simulink model "zcu216_tut_rfdc"  (R2019a)
settings: Solver=VariableStepDiscrete  StartTime=0.0  StopTime=10.0  RelTol=1e-3
undefined symbols (not defined in the file): es1, I, Q
libraries: xbsIndex_r4 x206, xps_library x3, casper_library_misc x1
(part 1 of 4)
settings Model: Creator=mcb  LastModifiedBy=mcb
settings OptimizationCC: DefaultParameterBehavior=Inlined

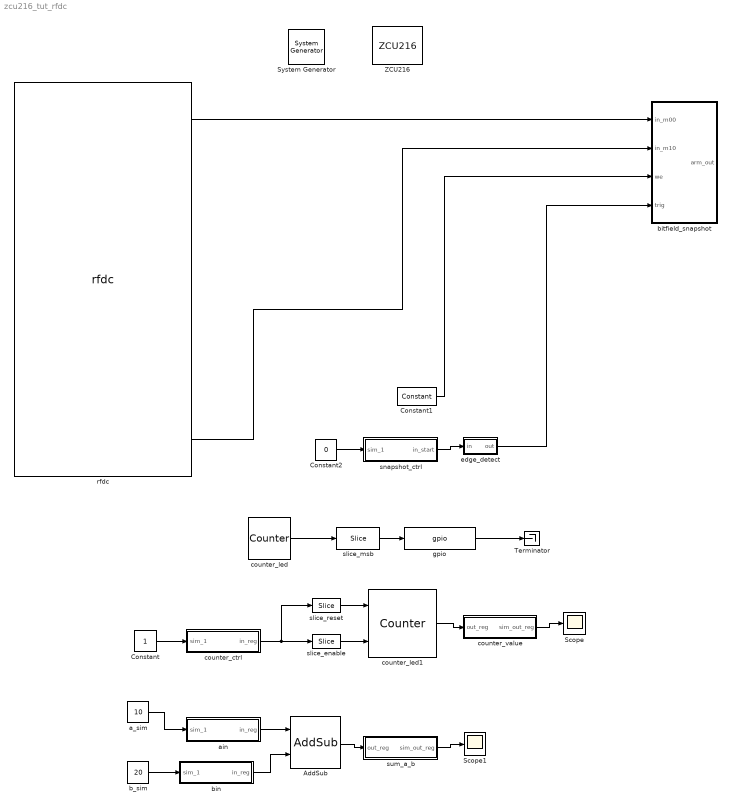
== system zcu216_tut_rfdc ==
  " System Generator" : xbsIndex_r4/ System Generator  Tag=genX  xilinxfamily=zynquplusRFSOCes1  part=xczu49dr  speed=-2-e-es1  package=ffvf1760  synthesis_tool=XST  clock_wrapper=Clock Enables  directory=/home/mcb/git/casper/tutorials_devel/rfsoc/tut_rfdc/zcu216_tut_rfdc/sysgen  proj_type=Vivado  Synth_file=Vivado Synthesis Defaults  Impl_file=Vivado Implementation Defaults  testbench=off  simulink_period=1  sysclk_period=4  dcm_input_clock_period=10  incr_netlist=off  trim_vbits=Everywhere in SubSystem  dbl_ovrd=According to Block Masks  core_generation=According to Block Masks  run_coregen=off  deprecated_control=off  eval_field=0  block_type=sysgen
  AddSub : xbsIndex_r4/AddSub  mode=Addition  use_carryin=off  use_carryout=off  en=off  latency=0  precision=User Defined  arith_type=Unsigned  n_bits=32  bin_pt=0  quantization=Truncate  overflow=Saturate  use_behavioral_HDL=off  hw_selection=Fabric  pipelined=off  dbl_ovrd=off  block_type=addsub
  Constant : Constant
  Constant1 : xbsIndex_r4/Constant  const=1.0  gui_display_data_type=Boolean  arith_type=Boolean  n_bits=16  bin_pt=14  preci_type=Single  exp_width=8  frac_width=24  explicit_period=on  period=1  equ=P=C  opselect=C  inp2=PCIN>>17  opr=+  inp1=P  carry=CIN  dbl_ovrd=off  block_type=constant
  Constant2 : Constant  Value=0
  Scope : Scope
  Scope1 : Scope
  Terminator : Terminator
  ZCU216 : xps_library/Platforms/ZCU216  Tag=xps:xsg  hw_sys=ZCU216:xczu49dr  clk_src=adc_clk  clk_rate=250  pl_clk_rate=125  sample_period=1  synthesis_tool=XST
      settings: SourceProductName=CASPER XPS Blockset
  a_sim : Constant  Value=10
  ain : Subsystem  Tag=xps:sw_reg  AncestorBlock=xps_library/Memory/software_register  mask(swreg){io_dir=From Processor, io_delay=0, init_val=0, sample_period=1, names=reg, bitwidths=32, bin_pts=0, arith_types=0, sim_port=on, show_format=off}
      mask prompts: io_dir "I/O direction"; io_delay "I/O delay"; init_val "Initial Value"; sample_period "Sample period"; names "Bitfield names [msb...lsb]"; bitwidths "Bitfield widths"; bin_pts "Bitfield binary pts"; arith_types "Bitfield types, ufix=0, fix=1, bool=2"; sim_port "Provide sim input/output?"; show_format "Print format string?"
      mask help: A 32-bit software-accessible register. Can be divided into bitfields of varying widths and types using the fields in the block mask.
      mask init:
      | swreg_init(gcb)
      settings: AttributesFormatString=1input
      mask TypeOptions io_dir: To Processor | From Processor
      mask Callback io_dir:
      | mask_enables = get_param(gcb, 'MaskEnables');
      | mask_names = get_param(gcb, 'MaskNames');
      | if strcmp(get_param(gcb, 'io_dir'), 'To Processor'),
      |     mask_enables{ismember(mask_names, 'sample_period')} = 'off';
      | else
      |     mask_enables{ismember(mask_names, 'sample_period')} = 'on';
      | end
      | set_param(gcb, 'MaskEnables', mask_enables);
      mask DialogControl ParameterTabVar0 Prompt: Setup
  b_sim : Constant  Value=20
  bin : Subsystem  Tag=xps:sw_reg  AncestorBlock=xps_library/Memory/software_register  mask(swreg){io_dir=From Processor, io_delay=0, init_val=0, sample_period=1, names=reg, bitwidths=32, bin_pts=0, arith_types=0, sim_port=on, show_format=off}
      mask prompts: io_dir "I/O direction"; io_delay "I/O delay"; init_val "Initial Value"; sample_period "Sample period"; names "Bitfield names [msb...lsb]"; bitwidths "Bitfield widths"; bin_pts "Bitfield binary pts"; arith_types "Bitfield types, ufix=0, fix=1, bool=2"; sim_port "Provide sim input/output?"; show_format "Print format string?"
      mask help: A 32-bit software-accessible register. Can be divided into bitfields of varying widths and types using the fields in the block mask.
      mask init:
      | swreg_init(gcb)
      settings: AttributesFormatString=1input
      mask TypeOptions io_dir: To Processor | From Processor
      mask Callback io_dir:
      | mask_enables = get_param(gcb, 'MaskEnables');
      | mask_names = get_param(gcb, 'MaskNames');
      | if strcmp(get_param(gcb, 'io_dir'), 'To Processor'),
      |     mask_enables{ismember(mask_names, 'sample_period')} = 'off';
      | else
      |     mask_enables{ismember(mask_names, 'sample_period')} = 'on';
      | end
      | set_param(gcb, 'MaskEnables', mask_enables);
      mask DialogControl ParameterTabVar0 Prompt: Setup
  bitfield_snapshot : Subsystem  Tag=casper:bitsnap  AncestorBlock=casper_library_scopes/bitfield_snapshot  mask(bitsnap){io_names=[m00 m10], io_widths=[64 64], io_bps=[0 0], io_types=[1 1], show_format=on, snap_storage=bram, snap_dram_dimm=2, snap_dram_clock=250, snap_nsamples=14, snap_data_width=128, snap_offset=off, snap_circap=off, snap_value=off, snap_ext_arm=off, snap_ext_circ=off, snap_provide_outputs=on, snap_use_dsp48=on, snap_delay=2, extra_names=[c d], extra_widths=[30 2], extra_bps=[0 0], extra_types=[0 0]}
      mask prompts: io_names "Names [msb...lsb]"; io_widths "Bitwidths [msb...lsb]"; io_bps "Binary pts [msb...lsb]"; io_types "Data types [msb...lsb], ufix=0, fix=1, bool=2"; show_format "Print format string?"; snap_storage "Storage medium"; snap_dram_dimm "DRAM dimm"; snap_dram_clock "DRAM clock rate"; snap_nsamples "Number of Samples (2^?)"; snap_data_width "Data width"; snap_offset "Start delay support"; snap_circap "Circular capture support"; snap_value "Extra value capture support"; snap_ext_arm "External arm support"; snap_ext_circ "External circular capture support"; snap_provide_outputs "Provide outputs"; snap_use_dsp48 "Use DSP48s to implement counters"; snap_delay "Pre-snapshot delay"; extra_names "Names [msb...lsb]"; extra_widths "Widths [msb...lsb]"; extra_bps "Binary pts [msb...lsb]"; extra_types "Data types [msb...lsb], ufix=0, fix=1, bool=2"
      mask help:
      | A wrapped snapshot block. Allows specification of inputs to a snapblock word so the toolflow can automatically set up the scope.
      | See documentation for snapshot for explanation of parameters.
      mask init:
      | bitsnap_init(gcb);
      settings: AttributesFormatString=|
      | snap(2):f64.0,f64.0 = 128 bits\n128 wide, 16384 deep
      | debugID: 51089287
      mask TypeOptions snap_storage: bram | dram
      mask Callback snap_storage: bitsnap_callback();
      mask TypeOptions snap_dram_dimm: 1 | 2 | 3 | 4
      mask TypeOptions snap_dram_clock: 200 | 250 | 266 | 300 | 333
      mask TypeOptions snap_data_width: 8 | 16 | 32 | 64 | 128
      mask Callback snap_value: bitsnap_callback();
      mask Callback snap_ext_arm: bitsnap_callback();
      mask Callback snap_ext_circ: bitsnap_callback();
      mask Callback snap_provide_outputs: bitsnap_callback();
      mask DialogControl ParameterTabVar0 Prompt: Inputs
      mask DialogControl ParameterTabVar01 Prompt: Snapshot
      mask DialogControl ParameterTabVar012 Prompt: Extra Value
  counter_ctrl : Subsystem  Tag=xps:sw_reg  AncestorBlock=xps_library/Memory/software_register  mask(swreg){io_dir=From Processor, io_delay=0, init_val=0, sample_period=1, names=reg, bitwidths=32, bin_pts=0, arith_types=0, sim_port=on, show_format=off}
      mask prompts: io_dir "I/O direction"; io_delay "I/O delay"; init_val "Initial Value"; sample_period "Sample period"; names "Bitfield names [msb...lsb]"; bitwidths "Bitfield widths"; bin_pts "Bitfield binary pts"; arith_types "Bitfield types, ufix=0, fix=1, bool=2"; sim_port "Provide sim input/output?"; show_format "Print format string?"
      mask help: A 32-bit software-accessible register. Can be divided into bitfields of varying widths and types using the fields in the block mask.
      mask init:
      | swreg_init(gcb)
      settings: AttributesFormatString=1input
      mask TypeOptions io_dir: To Processor | From Processor
      mask Callback io_dir:
      | mask_enables = get_param(gcb, 'MaskEnables');
      | mask_names = get_param(gcb, 'MaskNames');
      | if strcmp(get_param(gcb, 'io_dir'), 'To Processor'),
      |     mask_enables{ismember(mask_names, 'sample_period')} = 'off';
      | else
      |     mask_enables{ismember(mask_names, 'sample_period')} = 'on';
      | end
      | set_param(gcb, 'MaskEnables', mask_enables);
      mask DialogControl ParameterTabVar0 Prompt: Setup
  counter_led : xbsIndex_r4/Counter  cnt_type=Free Running  cnt_to=Inf  operation=Up  start_count=0  cnt_by_val=1  arith_type=Unsigned  n_bits=28  bin_pt=0  load_pin=off  rst=off  en=off  explicit_period=on  period=1  use_behavioral_HDL=off  implementation=Fabric  dbl_ovrd=off  block_type=counter
  counter_led1 : xbsIndex_r4/Counter  cnt_type=Free Running  cnt_to=Inf  operation=Up  start_count=0  cnt_by_val=1  arith_type=Unsigned  n_bits=32  bin_pt=0  load_pin=off  rst=on  en=on  explicit_period=on  period=1  use_behavioral_HDL=off  implementation=Fabric  dbl_ovrd=off  block_type=counter
  counter_value : Subsystem  Tag=xps:sw_reg  AncestorBlock=xps_library/Memory/software_register  mask(swreg){io_dir=To Processor, io_delay=0, init_val=0, sample_period=1, names=reg, bitwidths=32, bin_pts=0, arith_types=0, sim_port=on, show_format=off}
      mask prompts: io_dir "I/O direction"; io_delay "I/O delay"; init_val "Initial Value"; sample_period "Sample period"; names "Bitfield names [msb...lsb]"; bitwidths "Bitfield widths"; bin_pts "Bitfield binary pts"; arith_types "Bitfield types, ufix=0, fix=1, bool=2"; sim_port "Provide sim input/output?"; show_format "Print format string?"
      mask help: A 32-bit software-accessible register. Can be divided into bitfields of varying widths and types using the fields in the block mask.
      mask init:
      | swreg_init(gcb)
      settings: AttributesFormatString=1output
      mask TypeOptions io_dir: To Processor | From Processor
      mask Callback io_dir:
      | mask_enables = get_param(gcb, 'MaskEnables');
      | mask_names = get_param(gcb, 'MaskNames');
      | if strcmp(get_param(gcb, 'io_dir'), 'To Processor'),
      |     mask_enables{ismember(mask_names, 'sample_period')} = 'off';
      | else
      |     mask_enables{ismember(mask_names, 'sample_period')} = 'on';
      | end
      | set_param(gcb, 'MaskEnables', mask_enables);
      mask DialogControl ParameterTabVar0 Prompt: Setup
  edge_detect : Subsystem  AncestorBlock=casper_library_misc/edge_detect  mask(edge_detect){edge=Rising, polarity=Active High, x_in=[0 0.08 0.08 0.16 0.16 0.24 0.24 0.32 0.32 0.4], y_in=[-1 -1  1  1  1  1  1  1  1  1], x_out=[0.6 0.68 0.68 0.76 0.76 0.84 0.84 0.92 0.92 1], y_out=[-1 -1  1  1 -1 -1 -1 -1 -1 -1]}
      mask prompts: edge "Edge Type"; polarity "Output Polarity"; x_in "Input X Positions"; y_in "Input Y Positions"; x_out "Output X Positions"; y_out "Output Y Positions"
      mask help: Output is active for one-cycle after each edge of the specified type (i.e. rising, falling or both).
      mask init:
      | edge_detect_init(gcb,...
      |     'edge',edge,...
      |     'polarity',polarity,...
      |     'x_in',x_in,...
      |     'x_out',x_out,...
      |     'y_in',y_in,...
      |     'y_out',y_out);
      | 
      | x_in_num=str2num(getfield(getfield(get_param(gcb,'UserData'),'parameters'),'x_in'));
      | x_out_num=str2num(getfield(getfield(get_param(gcb,'UserData'),'parameters'),'x_out'));
      | y_in_num=str2num(getfield(getfield(get_param(gcb,'UserData'),'parameters'),'y_in'));
      | y_out_num=str2num(getfield(getfield(get_param(gcb,'UserData'),'parameters'),'y_out'));
      settings: AttributesFormatString=|
      | rising edges
      | active high
      mask Help: Output is active for one-cycle after each edge of the specified type (i.e. rising, falling, or both).  Latency is zero.
      mask TypeOptions edge: Rising | Falling | Both
      mask TypeOptions polarity: Active High | Active Low
      mask Display:
      | plot(x_in_num,0.5+y_in_num*0.2);
      | plot(x_out_num,0.5+y_out_num*0.2);
  gpio : xps_library/IO/gpio  Tag=xps:gpio  io_group_params_forwarded=on  io_group=ROACH2:led  io_group_real=led  io_group_custom=0  io_dir=out  arith_type=Boolean  bitwidth=1  bin_pt=0  bit_index=0  sample_period=1  use_single_ended=off  use_ddr=off  reg_iob=on  reg_clk_phase=0  termination=None
      settings: SourceProductName=CASPER XPS Blockset
  rfdc : xps_library/ADCs/rfdc  Tag=xps:rfdc  forceredraw=0  maskopening=1  runinit=1  Tile224_enable=on  t224_enable_mts=off  t224_sample_rate=2000  t224_clk_out=125  t224_enable_pll=on  t224_ref_clk=250  t224_QT_adc0_enable=on  t224_QT_adc0_digital_output=I/Q  t224_QT_adc0_dec_mode=4x  t224_QT_adc0_sample_per_cycle=4  t224_QT_adc0_req_axis_clk=250  t224_QT_adc0_mixer_type=Fine  t224_QT_adc0_mixer_mode=Real -> I/Q  t224_QT_adc0_nco_freq=0.5  t224_QT_adc0_nco_phase=0  t224_QT_adc0_coarse_freq=0  t224_QT_adc0_nyquist_zone=Zone 2  t224_QT_adc0_cal_mode=Mode 2  t224_QT_adc1_enable=off  t224_QT_adc1_digital_output=I/Q  t224_QT_adc1_dec_mode=4x  t224_QT_adc1_sample_per_cycle=4  t224_QT_adc1_req_axis_clk=250  t224_QT_adc1_mixer_type=Fine  t224_QT_adc1_mixer_mode=Real -> I/Q  t224_QT_adc1_nco_freq=0  t224_QT_adc1_nco_phase=0  t224_QT_adc1_coarse_freq=0  t224_QT_adc1_nyquist_zone=Zone 1  t224_QT_adc1_cal_mode=Mode 2  t224_QT_adc2_enable=on  t224_QT_adc2_digital_output=I/Q  t224_QT_adc2_dec_mode=4x  t224_QT_adc2_sample_per_cycle=4  t224_QT_adc2_req_axis_clk=250  t224_QT_adc2_mixer_type=Fine  t224_QT_adc2_mixer_mode=Real -> I/Q  t224_QT_adc2_nco_freq=0.5  t224_QT_adc2_nco_phase=0  t224_QT_adc2_coarse_freq=0  t224_QT_adc2_nyquist_zone=Zone 2  t224_QT_adc2_cal_mode=Mode 2  t224_QT_adc3_enable=off  t224_QT_adc3_digital_output=I/Q  t224_QT_adc3_dec_mode=4x  t224_QT_adc3_sample_per_cycle=4  t224_QT_adc3_req_axis_clk=250  t224_QT_adc3_mixer_type=Fine  t224_QT_adc3_mixer_mode=Real -> I/Q  t224_QT_adc3_nco_freq=0  t224_QT_adc3_nco_phase=0  t224_QT_adc3_coarse_freq=0  t224_QT_adc3_nyquist_zone=Zone 1  t224_QT_adc3_cal_mode=Mode 2  t224_DT_adc0_enable=on  t224_DT_adc0_digital_output=Real  t224_DT_adc0_dec_mode=2x  t224_DT_adc0_sample_per_cycle=8  t224_DT_adc0_req_axis_clk=125  t224_DT_adc0_mixer_type=Bypassed  t224_DT_adc0_mixer_mode=Real -> Real  t224_DT_adc0_nco_freq=0  t224_DT_adc0_nco_phase=0  t224_DT_adc0_coarse_freq=0  t224_DT_adc0_nyquist_zone=Zone 1  t224_DT_adc0_cal_mode=Mode 2  t224_DT_adc1_enable=on  t224_DT_adc1_digital_output=Real  t224_DT_adc1_dec_mode=2x  t224_DT_adc1_sample_per_cycle=8  t224_DT_adc1_req_axis_clk=125  t224_DT_adc1_mixer_type=Bypassed  t224_DT_adc1_mixer_mode=Real -> Real  t224_DT_adc1_nco_freq=0  t224_DT_adc1_nco_phase=0  t224_DT_adc1_coarse_freq=0  t224_DT_adc1_nyquist_zone=Zone 1  t224_DT_adc1_cal_mode=Mode 2  Tile225_enable=on  t225_enable_mts=off  t225_sample_rate=2000  t225_clk_out=125  t225_enable_pll=on  t225_ref_clk=250  t225_QT_adc0_enable=on  t225_QT_adc0_digital_output=I/Q  t225_QT_adc0_dec_mode=4x  t225_QT_adc0_sample_per_cycle=4  t225_QT_adc0_req_axis_clk=250  t225_QT_adc0_mixer_type=Bypassed  t225_QT_adc0_mixer_mode=Real -> Real  t225_QT_adc0_nco_freq=0.5  t225_QT_adc0_nco_phase=0  t225_QT_adc0_coarse_freq=0  t225_QT_adc0_nyquist_zone=Zone 2  t225_QT_adc0_cal_mode=Mode 2  t225_QT_adc1_enable=off  t225_QT_adc1_digital_output=Real  t225_QT_adc1_dec_mode=4x  t225_QT_adc1_sample_per_cycle=2  t225_QT_adc1_req_axis_clk=250  t225_QT_adc1_mixer_type=Bypassed  t225_QT_adc1_mixer_mode=Real -> Real  t225_QT_adc1_nco_freq=0  t225_QT_adc1_nco_phase=0  t225_QT_adc1_coarse_freq=0  t225_QT_adc1_nyquist_zone=Zone 1  t225_QT_adc1_cal_mode=Mode 2  t225_QT_adc2_enable=on  t225_QT_adc2_digital_output=I/Q  t225_QT_adc2_dec_mode=4x  t225_QT_adc2_sample_per_cycle=4  t225_QT_adc2_req_axis_clk=250  t225_QT_adc2_mixer_type=Bypassed  t225_QT_adc2_mixer_mode=Real -> Real  t225_QT_adc2_nco_freq=0.5  t225_QT_adc2_nco_phase=0  t225_QT_adc2_coarse_freq=0  t225_QT_adc2_nyquist_zone=Zone 2  t225_QT_adc2_cal_mode=Mode 2  t225_QT_adc3_enable=off  t225_QT_adc3_digital_output=Real  t225_QT_adc3_dec_mode=4x  t225_QT_adc3_sample_per_cycle=2  t225_QT_adc3_req_axis_clk=250  t225_QT_adc3_mixer_type=Bypassed  t225_QT_adc3_mixer_mode=Real -> Real  t225_QT_adc3_nco_freq=0  t225_QT_adc3_nco_phase=0  t225_QT_adc3_coarse_freq=0  t225_QT_adc3_nyquist_zone=Zone 1  t225_QT_adc3_cal_mode=Mode 2  t225_DT_adc0_enable=on  t225_DT_adc0_digital_output=Real  t225_DT_adc0_dec_mode=2x  t225_DT_adc0_sample_per_cycle=8  t225_DT_adc0_req_axis_clk=125  t225_DT_adc0_mixer_type=Bypassed  t225_DT_adc0_mixer_mode=Real -> Real  t225_DT_adc0_nco_freq=0  t225_DT_adc0_nco_phase=0  t225_DT_adc0_coarse_freq=0  t225_DT_adc0_nyquist_zone=Zone 1  t225_DT_adc0_cal_mode=Mode 2  t225_DT_adc1_enable=on  t225_DT_adc1_digital_output=Real  t225_DT_adc1_dec_mode=2x  t225_DT_adc1_sample_per_cycle=8  t225_DT_adc1_req_axis_clk=125  t225_DT_adc1_mixer_type=Bypassed  t225_DT_adc1_mixer_mode=Real -> Real  t225_DT_adc1_nco_freq=0  t225_DT_adc1_nco_phase=0  t225_DT_adc1_coarse_freq=0  t225_DT_adc1_nyquist_zone=Zone 1  t225_DT_adc1_cal_mode=Mode 2  Tile226_enable=on  t226_enable_mts=off  t226_sample_rate=2000  t226_clk_out=125  t226_enable_pll=on  t226_ref_clk=250  t226_QT_adc0_enable=on  t226_QT_adc0_digital_output=I/Q  t226_QT_adc0_dec_mode=4x  t226_QT_adc0_sample_per_cycle=4  t226_QT_adc0_req_axis_clk=250  t226_QT_adc0_mixer_type=Bypassed  t226_QT_adc0_mixer_mode=Real -> Real  t226_QT_adc0_nco_freq=0.5  t226_QT_adc0_nco_phase=0  t226_QT_adc0_coarse_freq=0  t226_QT_adc0_nyquist_zone=Zone 2  t226_QT_adc0_cal_mode=Mode 2  t226_QT_adc1_enable=off  t226_QT_adc1_digital_output=Real  t226_QT_adc1_dec_mode=4x  t226_QT_adc1_sample_per_cycle=2  t226_QT_adc1_req_axis_clk=250  t226_QT_adc1_mixer_type=Bypassed  t226_QT_adc1_mixer_mode=Real -> Real  t226_QT_adc1_nco_freq=0  t226_QT_adc1_nco_phase=0  t226_QT_adc1_coarse_freq=0  t226_QT_adc1_nyquist_zone=Zone 1  t226_QT_adc1_cal_mode=Mode 2  t226_QT_adc2_enable=off  t226_QT_adc2_digital_output=Real  t226_QT_adc2_dec_mode=4x  t226_QT_adc2_sample_per_cycle=2  t226_QT_adc2_req_axis_clk=250  t226_QT_adc2_mixer_type=Bypassed  t226_QT_adc2_mixer_mode=Real -> Real  t226_QT_adc2_nco_freq=0  t226_QT_adc2_nco_phase=0  t226_QT_adc2_coarse_freq=0  t226_QT_adc2_nyquist_zone=Zone 1  t226_QT_adc2_cal_mode=Mode 2  t226_QT_adc3_enable=off  t226_QT_adc3_digital_output=Real  t226_QT_adc3_dec_mode=4x  t226_QT_adc3_sample_per_cycle=2  t226_QT_adc3_req_axis_clk=250  t226_QT_adc3_mixer_type=Bypassed  t226_QT_adc3_mixer_mode=Real -> Real  t226_QT_adc3_nco_freq=0  t226_QT_adc3_nco_phase=0  t226_QT_adc3_coarse_freq=0  t226_QT_adc3_nyquist_zone=Zone 1  t226_QT_adc3_cal_mode=Mode 2  t226_DT_adc0_enable=on  t226_DT_adc0_digital_output=Real  t226_DT_adc0_dec_mode=2x  t226_DT_adc0_sample_per_cycle=8  t226_DT_adc0_req_axis_clk=125  t226_DT_adc0_mixer_type=Bypassed  t226_DT_adc0_mixer_mode=Real -> Real  t226_DT_adc0_nco_freq=0  t226_DT_adc0_nco_phase=0  t226_DT_adc0_coarse_freq=0  t226_DT_adc0_nyquist_zone=Zone 1  t226_DT_adc0_cal_mode=Mode 2  t226_DT_adc1_enable=on  t226_DT_adc1_digital_output=Real  t226_DT_adc1_dec_mode=2x  t226_DT_adc1_sample_per_cycle=8  t226_DT_adc1_req_axis_clk=125  t226_DT_adc1_mixer_type=Bypassed  t226_DT_adc1_mixer_mode=Real -> Real  t226_DT_adc1_nco_freq=0  t226_DT_adc1_nco_phase=0  t226_DT_adc1_coarse_freq=0  t226_DT_adc1_nyquist_zone=Zone 1  t226_DT_adc1_cal_mode=Mode 2  Tile227_enable=on  t227_enable_mts=off  t227_sample_rate=2000  t227_clk_out=125  t227_enable_pll=on  t227_ref_clk=250  t227_QT_adc0_enable=on  t227_QT_adc0_digital_output=I/Q  t227_QT_adc0_dec_mode=4x  t227_QT_adc0_sample_per_cycle=4  t227_QT_adc0_req_axis_clk=250  t227_QT_adc0_mixer_type=Bypassed  t227_QT_adc0_mixer_mode=Real -> Real  t227_QT_adc0_nco_freq=0.5  t227_QT_adc0_nco_phase=0  t227_QT_adc0_coarse_freq=0  t227_QT_adc0_nyquist_zone=Zone 2  t227_QT_adc0_cal_mode=Mode 2  t227_QT_adc1_enable=off  t227_QT_adc1_digital_output=Real  t227_QT_adc1_dec_mode=4x  t227_QT_adc1_sample_per_cycle=2  t227_QT_adc1_req_axis_clk=250  t227_QT_adc1_mixer_type=Bypassed  t227_QT_adc1_mixer_mode=Real -> Real  t227_QT_adc1_nco_freq=0  t227_QT_adc1_nco_phase=0  t227_QT_adc1_coarse_freq=0  t227_QT_adc1_nyquist_zone=Zone 1  t227_QT_adc1_cal_mode=Mode 2  t227_QT_adc2_enable=off  t227_QT_adc2_digital_output=Real  t227_QT_adc2_dec_mode=4x  t227_QT_adc2_sample_per_cycle=2  t227_QT_adc2_req_axis_clk=250  t227_QT_adc2_mixer_type=Bypassed  t227_QT_adc2_mixer_mode=Real -> Real  t227_QT_adc2_nco_freq=0  t227_QT_adc2_nco_phase=0  t227_QT_adc2_coarse_freq=0  t227_QT_adc2_nyquist_zone=Zone 1  t227_QT_adc2_cal_mode=Mode 2  t227_QT_adc3_enable=off  t227_QT_adc3_digital_output=Real  t227_QT_adc3_dec_mode=4x  t227_QT_adc3_sample_per_cycle=2  t227_QT_adc3_req_axis_clk=250  t227_QT_adc3_mixer_type=Bypassed  t227_QT_adc3_mixer_mode=Real -> Real  t227_QT_adc3_nco_freq=0  t227_QT_adc3_nco_phase=0  t227_QT_adc3_coarse_freq=0  t227_QT_adc3_nyquist_zone=Zone 1  t227_QT_adc3_cal_mode=Mode 2  t227_DT_adc0_enable=on  t227_DT_adc0_digital_output=Real  t227_DT_adc0_dec_mode=2x  t227_DT_adc0_sample_per_cycle=8  t227_DT_adc0_req_axis_clk=125  t227_DT_adc0_mixer_type=Bypassed  t227_DT_adc0_mixer_mode=Real -> Real  t227_DT_adc0_nco_freq=0  t227_DT_adc0_nco_phase=0  t227_DT_adc0_coarse_freq=0  t227_DT_adc0_nyquist_zone=Zone 1  t227_DT_adc0_cal_mode=Mode 2  t227_DT_adc1_enable=on  t227_DT_adc1_digital_output=Real  t227_DT_adc1_dec_mode=2x  t227_DT_adc1_sample_per_cycle=8  t227_DT_adc1_req_axis_clk=125  t227_DT_adc1_mixer_type=Bypassed  t227_DT_adc1_mixer_mode=Real -> Real  t227_DT_adc1_nco_freq=0  t227_DT_adc1_nco_phase=0  t227_DT_adc1_coarse_freq=0  t227_DT_adc1_nyquist_zone=Zone 1  t227_DT_adc1_cal_mode=Mode 2  Tile228_enable=off  t228_enable_mts=off  t228_sample_rate=2000  t228_clk_out=125  t228_enable_pll=on  t228_ref_clk=250  t228_output_power=20  t228_QT_dac0_enable=off  t228_QT_dac0_analog_output=Real  t228_QT_dac0_inter_mode=4x  t228_QT_dac0_sample_per_cycle=2  t228_QT_dac0_req_axis_clk=250  t228_QT_dac0_datapath_mode=DUC 0 to Fs/2  t228_QT_dac0_mixer_type=Bypassed  t228_QT_dac0_mixer_mode=Real -> Real  t228_QT_dac0_nco_freq=0  t228_QT_dac0_nco_phase=0  t228_QT_dac0_coarse_freq=0  t228_QT_dac0_nyquist_zone=Zone 1  t228_QT_dac0_decode_mode=SNR Optimized  t228_QT_dac1_enable=off  t228_QT_dac1_analog_output=Real  t228_QT_dac1_inter_mode=4x  t228_QT_dac1_sample_per_cycle=2  t228_QT_dac1_req_axis_clk=250  t228_QT_dac1_datapath_mode=DUC 0 to Fs/2  t228_QT_dac1_mixer_type=Bypassed  t228_QT_dac1_mixer_mode=Real -> Real  t228_QT_dac1_nco_freq=0  t228_QT_dac1_nco_phase=0  t228_QT_dac1_coarse_freq=0  t228_QT_dac1_nyquist_zone=Zone 1  t228_QT_dac1_decode_mode=SNR Optimized  t228_QT_dac2_enable=off  t228_QT_dac2_analog_output=Real  t228_QT_dac2_inter_mode=4x  t228_QT_dac2_sample_per_cycle=2  t228_QT_dac2_req_axis_clk=250  t228_QT_dac2_datapath_mode=DUC 0 to Fs/2  t228_QT_dac2_mixer_type=Bypassed  t228_QT_dac2_mixer_mode=Real -> Real  t228_QT_dac2_nco_freq=0  t228_QT_dac2_nco_phase=0  t228_QT_dac2_coarse_freq=0  t228_QT_dac2_nyquist_zone=Zone 1  t228_QT_dac2_decode_mode=SNR Optimized  t228_QT_dac3_enable=off  t228_QT_dac3_analog_output=Real  t228_QT_dac3_inter_mode=4x  t228_QT_dac3_sample_per_cycle=2  t228_QT_dac3_req_axis_clk=250  t228_QT_dac3_datapath_mode=DUC 0 to Fs/2  t228_QT_dac3_mixer_type=Bypassed  t228_QT_dac3_mixer_mode=Real -> Real  t228_QT_dac3_nco_freq=0  t228_QT_dac3_nco_phase=0  t228_QT_dac3_coarse_freq=0  t228_QT_dac3_nyquist_zone=Zone 1  t228_QT_dac3_decode_mode=SNR Optimized  t228_DT_dac0_enable=on  t228_DT_dac0_analog_output=I/Q  t228_DT_dac0_inter_mode=2x  t228_DT_dac0_sample_per_cycle=8  t228_DT_dac0_req_axis_clk=125  t228_DT_dac0_mixer_type=Fine  t228_DT_dac0_mixer_mode=I/Q -> I/Q  t228_DT_dac0_nco_freq=0  t228_DT_dac0_nco_phase=0  t228_DT_dac0_coarse_freq=0  t228_DT_dac0_nyquist_zone=Zone 1  t228_DT_dac0_decode_mode=SNR Optimized  t228_DT_dac1_enable=on  t228_DT_dac1_analog_output=I/Q  t228_DT_dac1_inter_mode=2x  t228_DT_dac1_sample_per_cycle=8  t228_DT_dac1_req_axis_clk=125  t228_DT_dac1_mixer_type=Off  t228_DT_dac1_mixer_mode=Off  t228_DT_dac1_nco_freq=0  t228_DT_dac1_nco_phase=0  t228_DT_dac1_coarse_freq=0  t228_DT_dac1_nyquist_zone=Zone 1  t228_DT_dac1_decode_mode=SNR Optimized  t228_DT_dac2_enable=on  t228_DT_dac2_analog_output=Real  t228_DT_dac2_inter_mode=2x  t228_DT_dac2_sample_per_cycle=8  t228_DT_dac2_req_axis_clk=125  t228_DT_dac2_mixer_type=Bypassed  t228_DT_dac2_mixer_mode=Real -> Real  t228_DT_dac2_nco_freq=0  t228_DT_dac2_nco_phase=0  t228_DT_dac2_coarse_freq=0  t228_DT_dac2_nyquist_zone=Zone 1  t228_DT_dac2_decode_mode=SNR Optimized  t228_DT_dac3_enable=off  t228_DT_dac3_analog_output=Real  t228_DT_dac3_inter_mode=2x  t228_DT_dac3_sample_per_cycle=8  t228_DT_dac3_req_axis_clk=125  t228_DT_dac3_mixer_type=Bypassed  t228_DT_dac3_mixer_mode=Real -> Real  t228_DT_dac3_nco_freq=0  t228_DT_dac3_nco_phase=0  t228_DT_dac3_coarse_freq=0  t228_DT_dac3_nyquist_zone=Zone 1  t228_DT_dac3_decode_mode=SNR Optimized  Tile229_enable=off  t229_enable_mts=off  t229_sample_rate=2000  t229_clk_out=125  t229_enable_pll=on  t229_ref_clk=250  t229_output_power=20  t229_QT_dac0_enable=off  t229_QT_dac0_analog_output=Real  t229_QT_dac0_inter_mode=4x  t229_QT_dac0_sample_per_cycle=2  t229_QT_dac0_req_axis_clk=250  t229_QT_dac0_datapath_mode=DUC 0 to Fs/2  t229_QT_dac0_mixer_type=Bypassed  t229_QT_dac0_mixer_mode=Real -> Real  t229_QT_dac0_nco_freq=0  t229_QT_dac0_nco_phase=0  t229_QT_dac0_coarse_freq=0  t229_QT_dac0_nyquist_zone=Zone 1  t229_QT_dac0_decode_mode=SNR Optimized  t229_QT_dac1_enable=off  t229_QT_dac1_analog_output=Real  t229_QT_dac1_inter_mode=4x  t229_QT_dac1_sample_per_cycle=2  t229_QT_dac1_req_axis_clk=250  t229_QT_dac1_datapath_mode=DUC 0 to Fs/2  t229_QT_dac1_mixer_type=Bypassed  t229_QT_dac1_mixer_mode=Real -> Real  t229_QT_dac1_nco_freq=0  t229_QT_dac1_nco_phase=0  t229_QT_dac1_coarse_freq=0  t229_QT_dac1_nyquist_zone=Zone 1  t229_QT_dac1_decode_mode=SNR Optimized  t229_QT_dac2_enable=off  t229_QT_dac2_analog_output=Real  t229_QT_dac2_inter_mode=4x  t229_QT_dac2_sample_per_cycle=2  t229_QT_dac2_req_axis_clk=250  t229_QT_dac2_datapath_mode=DUC 0 to Fs/2  t229_QT_dac2_mixer_type=Bypassed  t229_QT_dac2_mixer_mode=Real -> Real  t229_QT_dac2_nco_freq=0  t229_QT_dac2_nco_phase=0  t229_QT_dac2_coarse_freq=0  t229_QT_dac2_nyquist_zone=Zone 1  t229_QT_dac2_decode_mode=SNR Optimized  t229_QT_dac3_enable=off  t229_QT_dac3_analog_output=Real  t229_QT_dac3_inter_mode=4x  t229_QT_dac3_sample_per_cycle=2  t229_QT_dac3_req_axis_clk=250  t229_QT_dac3_datapath_mode=DUC 0 to Fs/2  t229_QT_dac3_mixer_type=Bypassed  t229_QT_dac3_mixer_mode=Real -> Real  t229_QT_dac3_nco_freq=0  t229_QT_dac3_nco_phase=0  t229_QT_dac3_coarse_freq=0  t229_QT_dac3_nyquist_zone=Zone 1  t229_QT_dac3_decode_mode=SNR Optimized  t229_DT_dac0_enable=off  t229_DT_dac0_analog_output=Real  t229_DT_dac0_inter_mode=2x  t229_DT_dac0_sample_per_cycle=8  t229_DT_dac0_req_axis_clk=125  t229_DT_dac0_mixer_type=Bypassed  t229_DT_dac0_mixer_mode=Real -> Real  t229_DT_dac0_nco_freq=0  t229_DT_dac0_nco_phase=0  t229_DT_dac0_coarse_freq=0  t229_DT_dac0_nyquist_zone=Zone 1  t229_DT_dac0_decode_mode=SNR Optimized  t229_DT_dac1_enable=off  t229_DT_dac1_analog_output=Real  t229_DT_dac1_inter_mode=2x  t229_DT_dac1_sample_per_cycle=8  t229_DT_dac1_req_axis_clk=125  t229_DT_dac1_mixer_type=Bypassed  t229_DT_dac1_mixer_mode=Real -> Real  t229_DT_dac1_nco_freq=0  t229_DT_dac1_nco_phase=0  t229_DT_dac1_coarse_freq=0  t229_DT_dac1_nyquist_zone=Zone 1  t229_DT_dac1_decode_mode=SNR Optimized  t229_DT_dac2_enable=off  t229_DT_dac2_analog_output=Real  t229_DT_dac2_inter_mode=2x  t229_DT_dac2_sample_per_cycle=8  t229_DT_dac2_req_axis_clk=125  t229_DT_dac2_mixer_type=Bypassed  t229_DT_dac2_mixer_mode=Real -> Real  t229_DT_dac2_nco_freq=0  t229_DT_dac2_nco_phase=0  t229_DT_dac2_coarse_freq=0  t229_DT_dac2_nyquist_zone=Zone 1  t229_DT_dac2_decode_mode=SNR Optimized  t229_DT_dac3_enable=off  t229_DT_dac3_analog_output=Real  t229_DT_dac3_inter_mode=2x  t229_DT_dac3_sample_per_cycle=8  t229_DT_dac3_req_axis_clk=125  t229_DT_dac3_mixer_type=Bypassed  t229_DT_dac3_mixer_mode=Real -> Real  t229_DT_dac3_nco_freq=0  t229_DT_dac3_nco_phase=0  t229_DT_dac3_coarse_freq=0  t229_DT_dac3_nyquist_zone=Zone 1  t229_DT_dac3_decode_mode=SNR Optimized  Tile230_enable=off  t230_enable_mts=off  t230_sample_rate=2000  t230_clk_out=125  t230_enable_pll=on  t230_ref_clk=250  t230_output_power=20  t230_QT_dac0_enable=off  t230_QT_dac0_analog_output=Real  t230_QT_dac0_inter_mode=4x  t230_QT_dac0_sample_per_cycle=2  t230_QT_dac0_req_axis_clk=250  t230_QT_dac0_datapath_mode=DUC 0 to Fs/2  t230_QT_dac0_mixer_type=Bypassed  t230_QT_dac0_mixer_mode=Real -> Real  t230_QT_dac0_nco_freq=0  t230_QT_dac0_nco_phase=0  t230_QT_dac0_coarse_freq=0  t230_QT_dac0_nyquist_zone=Zone 1  t230_QT_dac0_decode_mode=SNR Optimized  t230_QT_dac1_enable=off  t230_QT_dac1_analog_output=Real  t230_QT_dac1_inter_mode=4x  t230_QT_dac1_sample_per_cycle=2  t230_QT_dac1_req_axis_clk=250  t230_QT_dac1_datapath_mode=DUC 0 to Fs/2  t230_QT_dac1_mixer_type=Bypassed  t230_QT_dac1_mixer_mode=Real -> Real  t230_QT_dac1_nco_freq=0  t230_QT_dac1_nco_phase=0  t230_QT_dac1_coarse_freq=0  t230_QT_dac1_nyquist_zone=Zone 1  t230_QT_dac1_decode_mode=SNR Optimized  t230_QT_dac2_enable=off  t230_QT_dac2_analog_output=Real  t230_QT_dac2_inter_mode=4x  t230_QT_dac2_sample_per_cycle=2  t230_QT_dac2_req_axis_clk=250  t230_QT_dac2_datapath_mode=DUC 0 to Fs/2  t230_QT_dac2_mixer_type=Bypassed  t230_QT_dac2_mixer_mode=Real -> Real  t230_QT_dac2_nco_freq=0  t230_QT_dac2_nco_phase=0  t230_QT_dac2_coarse_freq=0  t230_QT_dac2_nyquist_zone=Zone 1  t230_QT_dac2_decode_mode=SNR Optimized  t230_QT_dac3_enable=off  t230_QT_dac3_analog_output=Real  t230_QT_dac3_inter_mode=4x  t230_QT_dac3_sample_per_cycle=2  t230_QT_dac3_req_axis_clk=250  t230_QT_dac3_datapath_mode=DUC 0 to Fs/2  t230_QT_dac3_mixer_type=Bypassed  t230_QT_dac3_mixer_mode=Real -> Real  t230_QT_dac3_nco_freq=0  t230_QT_dac3_nco_phase=0  t230_QT_dac3_coarse_freq=0  t230_QT_dac3_nyquist_zone=Zone 1  t230_QT_dac3_decode_mode=SNR Optimized  Tile231_enable=off  t231_enable_mts=off  t231_sample_rate=2000  t231_clk_out=125  t231_enable_pll=on  t231_ref_clk=250  t231_output_power=20  t231_QT_dac0_enable=off  t231_QT_dac0_analog_output=Real  t231_QT_dac0_inter_mode=4x  t231_QT_dac0_sample_per_cycle=2  t231_QT_dac0_req_axis_clk=250  t231_QT_dac0_datapath_mode=DUC 0 to Fs/2  t231_QT_dac0_mixer_type=Bypassed  t231_QT_dac0_mixer_mode=Real -> Real  t231_QT_dac0_nco_freq=0  t231_QT_dac0_nco_phase=0  t231_QT_dac0_coarse_freq=0  t231_QT_dac0_nyquist_zone=Zone 1  t231_QT_dac0_decode_mode=SNR Optimized  t231_QT_dac1_enable=off  t231_QT_dac1_analog_output=Real  t231_QT_dac1_inter_mode=4x  t231_QT_dac1_sample_per_cycle=2  t231_QT_dac1_req_axis_clk=250  t231_QT_dac1_datapath_mode=DUC 0 to Fs/2  t231_QT_dac1_mixer_type=Bypassed  t231_QT_dac1_mixer_mode=Real -> Real  t231_QT_dac1_nco_freq=0  t231_QT_dac1_nco_phase=0  t231_QT_dac1_coarse_freq=0  t231_QT_dac1_nyquist_zone=Zone 1  t231_QT_dac1_decode_mode=SNR Optimized  t231_QT_dac2_enable=off  t231_QT_dac2_analog_output=Real  t231_QT_dac2_inter_mode=4x  t231_QT_dac2_sample_per_cycle=2  t231_QT_dac2_req_axis_clk=250  t231_QT_dac2_datapath_mode=DUC 0 to Fs/2  t231_QT_dac2_mixer_type=Bypassed  t231_QT_dac2_mixer_mode=Real -> Real  t231_QT_dac2_nco_freq=0  t231_QT_dac2_nco_phase=0  t231_QT_dac2_coarse_freq=0  t231_QT_dac2_nyquist_zone=Zone 1  t231_QT_dac2_decode_mode=SNR Optimized  t231_QT_dac3_enable=off  t231_QT_dac3_analog_output=Real  t231_QT_dac3_inter_mode=4x  t231_QT_dac3_sample_per_cycle=2  t231_QT_dac3_req_axis_clk=250  t231_QT_dac3_datapath_mode=DUC 0 to Fs/2  t231_QT_dac3_mixer_type=Bypassed  t231_QT_dac3_mixer_mode=Real -> Real  t231_QT_dac3_nco_freq=0  t231_QT_dac3_nco_phase=0  t231_QT_dac3_coarse_freq=0  t231_QT_dac3_nyquist_zone=Zone 1  t231_QT_dac3_decode_mode=SNR Optimized  t224_has_adc_clk=off  t224_adc_clk_src=226  t224_clk_dist=None  t225_has_adc_clk=on  t225_adc_clk_src=226  t225_clk_dist=None  t226_has_adc_clk=on  t226_adc_clk_src=226  t226_clk_dist=Input Refclk  t227_has_adc_clk=off  t227_adc_clk_src=226  t227_clk_dist=None  t228_has_dac_clk=off  t228_dac_clk_src=230  t228_clk_dist=None  t229_has_dac_clk=on  t229_dac_clk_src=230  t229_clk_dist=None  t230_has_dac_clk=on  t230_dac_clk_src=230  t230_clk_dist=Input Refclk  t231_has_dac_clk=off  t231_dac_clk_src=230  t231_clk_dist=None  maskdoneopening=0
      settings: SourceProductName=CASPER XPS Blockset
  slice_enable : xbsIndex_r4/Slice  nbits=1  boolean_output=on  mode=Lower Bit Location + Width  bit1=0  base1=MSB of Input  bit0=0  base0=LSB of Input  dbl_ovrd=off  block_type=slice
  slice_msb : xbsIndex_r4/Slice  nbits=1  boolean_output=off  mode=Upper Bit Location + Width  bit1=0  base1=MSB of Input  bit0=0  base0=LSB of Input  dbl_ovrd=off  block_type=slice
  slice_reset : xbsIndex_r4/Slice  nbits=1  boolean_output=on  mode=Lower Bit Location + Width  bit1=0  base1=MSB of Input  bit0=1  base0=LSB of Input  dbl_ovrd=off  block_type=slice
  snapshot_ctrl : Subsystem  Tag=xps:sw_reg  AncestorBlock=xps_library/Memory/software_register  mask(swreg){io_dir=From Processor, io_delay=0, init_val=0, sample_period=1, names=[start], bitwidths=1, bin_pts=0, arith_types=2, sim_port=on, show_format=on}
      mask prompts: io_dir "I/O direction"; io_delay "I/O delay"; init_val "Initial Value"; sample_period "Sample period"; names "Bitfield names [msb...lsb]"; bitwidths "Bitfield widths"; bin_pts "Bitfield binary pts"; arith_types "Bitfield types, ufix=0, fix=1, bool=2"; sim_port "Provide sim input/output?"; show_format "Print format string?"
      mask help: A 32-bit software-accessible register. Can be divided into bitfields of varying widths and types using the fields in the block mask.
      mask init:
      | swreg_init(gcb)
      settings: AttributesFormatString=1input:b = 1 bits
      mask TypeOptions io_dir: To Processor | From Processor
      mask Callback io_dir:
      | mask_enables = get_param(gcb, 'MaskEnables');
      | mask_names = get_param(gcb, 'MaskNames');
      | if strcmp(get_param(gcb, 'io_dir'), 'To Processor'),
      |     mask_enables{ismember(mask_names, 'sample_period')} = 'off';
      | else
      |     mask_enables{ismember(mask_names, 'sample_period')} = 'on';
      | end
      | set_param(gcb, 'MaskEnables', mask_enables);
      mask DialogControl ParameterTabVar0 Prompt: Setup
  sum_a_b : Subsystem  Tag=xps:sw_reg  AncestorBlock=xps_library/Memory/software_register  mask(swreg){io_dir=To Processor, io_delay=0, init_val=0, sample_period=1, names=reg, bitwidths=32, bin_pts=0, arith_types=0, sim_port=on, show_format=off}
      mask prompts: io_dir "I/O direction"; io_delay "I/O delay"; init_val "Initial Value"; sample_period "Sample period"; names "Bitfield names [msb...lsb]"; bitwidths "Bitfield widths"; bin_pts "Bitfield binary pts"; arith_types "Bitfield types, ufix=0, fix=1, bool=2"; sim_port "Provide sim input/output?"; show_format "Print format string?"
      mask help: A 32-bit software-accessible register. Can be divided into bitfields of varying widths and types using the fields in the block mask.
      mask init:
      | swreg_init(gcb)
      settings: AttributesFormatString=1output
      mask TypeOptions io_dir: To Processor | From Processor
      mask Callback io_dir:
      | mask_enables = get_param(gcb, 'MaskEnables');
      | mask_names = get_param(gcb, 'MaskNames');
      | if strcmp(get_param(gcb, 'io_dir'), 'To Processor'),
      |     mask_enables{ismember(mask_names, 'sample_period')} = 'off';
      | else
      |     mask_enables{ismember(mask_names, 'sample_period')} = 'on';
      | end
      | set_param(gcb, 'MaskEnables', mask_enables);
      mask DialogControl ParameterTabVar0 Prompt: Setup
  wires:
  b_sim/1 -> bin/1(sim_1)
  counter_value/1(sim_out_reg) -> Scope/1
  counter_ctrl/1(in_reg) -> slice_reset/1, slice_enable/1
  bin/1(in_reg) -> AddSub/2
  sum_a_b/1(sim_out_reg) -> Scope1/1
  counter_led/1 -> slice_msb/1
  slice_enable/1 -> counter_led1/2
  Constant2/1 -> snapshot_ctrl/1(sim_1)
  snapshot_ctrl/1(in_start) -> edge_detect/1(in)
  slice_reset/1 -> counter_led1/1
  gpio/1 -> Terminator/1
  Constant/1 -> counter_ctrl/1(sim_1)
  counter_led1/1 -> counter_value/1(out_reg)
  slice_msb/1 -> gpio/1
  AddSub/1 -> sum_a_b/1(out_reg)
  Constant1/1 -> bitfield_snapshot/3(we)
  edge_detect/1(out) -> bitfield_snapshot/4(trig)
  rfdc/1 -> bitfield_snapshot/1(in_m00)
  a_sim/1 -> ain/1(sim_1)
  ain/1(in_reg) -> AddSub/1
  rfdc/6 -> bitfield_snapshot/2(in_m10)

== system zcu216_tut_rfdc/ain ==
  sim_1 : Inport
  convert1_1 : DataTypeConversion  OutDataTypeStr=fixdt('ufix32_En0')  LockScale=on
  convert2_1 : DataTypeConversion  OutDataTypeStr=fixdt('ufix32_En0')  ConvertRealWorld=Stored Integer (SI)  LockScale=on
  gain_1 : Gain
  io_delay : xbsIndex_r4/Delay  rst=off  infoeditControl=Selection of Reset will increase slice count due to use of real FFs and instead of SRLs  en=off  latency=0  reg_retiming=on  dbl_ovrd=off  block_type=delay
  reint1 : xbsIndex_r4/Reinterpret  force_arith_type=on  arith_type=Unsigned  force_bin_pt=on  bin_pt=0  block_type=reinterpret
  slice_reg : xbsIndex_r4/Slice  nbits=32  boolean_output=off  mode=Lower Bit Location + Width  bit1=0  base1=MSB of Input  bit0=0  base0=LSB of Input  dbl_ovrd=off  block_type=slice
  zcu216_tut_rfdc_ain_user_data_out : xbsIndex_r4/Gateway In  gui_display_data_type=Fixed-point  arith_type=Unsigned  n_bits=32  bin_pt=0  preci_type=Single  exp_width=8  frac_width=24  rows=1  columns=1  quantization="Round  (unbiased: +/- Inf)"  overflow=Saturate  period=1  UseAsADC=off  ADCChannel='1'  interface=None  automatic_assignment=on  address_offset=hex2dec('00')  intf_name=''  intf_description=''  default_value=0  timing_constraint=None  locs_specified=off  LOCs={}  io_standard={}  inherit_from_input=off  hdl_port=on  dbl_ovrd=off  block_type=gatewayin
  in_reg : Outport  VectorParamsAs1DForOutWhenUnconnected=on
  wires:
  zcu216_tut_rfdc_ain_user_data_out/1 -> io_delay/1
  sim_1/1 -> convert1_1/1
  convert1_1/1 -> convert2_1/1
  convert2_1/1 -> gain_1/1
  gain_1/1 -> zcu216_tut_rfdc_ain_user_data_out/1
  io_delay/1 -> slice_reg/1
  slice_reg/1 -> reint1/1
  reint1/1 -> in_reg/1

== system zcu216_tut_rfdc/bin ==
  sim_1 : Inport
  convert1_1 : DataTypeConversion  OutDataTypeStr=fixdt('ufix32_En0')  LockScale=on
  convert2_1 : DataTypeConversion  OutDataTypeStr=fixdt('ufix32_En0')  ConvertRealWorld=Stored Integer (SI)  LockScale=on
  gain_1 : Gain
  io_delay : xbsIndex_r4/Delay  rst=off  infoeditControl=Selection of Reset will increase slice count due to use of real FFs and instead of SRLs  en=off  latency=0  reg_retiming=on  dbl_ovrd=off  block_type=delay
  reint1 : xbsIndex_r4/Reinterpret  force_arith_type=on  arith_type=Unsigned  force_bin_pt=on  bin_pt=0  block_type=reinterpret
  slice_reg : xbsIndex_r4/Slice  nbits=32  boolean_output=off  mode=Lower Bit Location + Width  bit1=0  base1=MSB of Input  bit0=0  base0=LSB of Input  dbl_ovrd=off  block_type=slice
  zcu216_tut_rfdc_bin_user_data_out : xbsIndex_r4/Gateway In  gui_display_data_type=Fixed-point  arith_type=Unsigned  n_bits=32  bin_pt=0  preci_type=Single  exp_width=8  frac_width=24  rows=1  columns=1  quantization="Round  (unbiased: +/- Inf)"  overflow=Saturate  period=1  UseAsADC=off  ADCChannel='1'  interface=None  automatic_assignment=on  address_offset=hex2dec('00')  intf_name=''  intf_description=''  default_value=0  timing_constraint=None  locs_specified=off  LOCs={}  io_standard={}  inherit_from_input=off  hdl_port=on  dbl_ovrd=off  block_type=gatewayin
  in_reg : Outport  VectorParamsAs1DForOutWhenUnconnected=on
  wires:
  zcu216_tut_rfdc_bin_user_data_out/1 -> io_delay/1
  sim_1/1 -> convert1_1/1
  convert1_1/1 -> convert2_1/1
  convert2_1/1 -> gain_1/1
  gain_1/1 -> zcu216_tut_rfdc_bin_user_data_out/1
  io_delay/1 -> slice_reg/1
  slice_reg/1 -> reint1/1
  reint1/1 -> in_reg/1

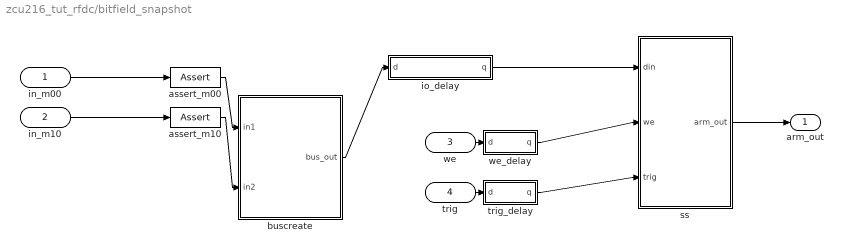
== system zcu216_tut_rfdc/bitfield_snapshot ==
  in_m00 : Inport
  in_m10 : Inport  Port=2
  we : Inport  Port=3
  trig : Inport  Port=4
  assert_m00 : xbsIndex_r4/Assert  assert_type=on  type_source=Explicitly  gui_display_data_type=Fixed-point  arith_type="Signed  (2's comp)"  n_bits=64  bin_pt=0  preci_type=Single  exp_width=8  frac_width=24  assert_rate=off  rate_source=Explicitly  period=1  output_port=on  block_type=assert
  assert_m10 : xbsIndex_r4/Assert  assert_type=on  type_source=Explicitly  gui_display_data_type=Fixed-point  arith_type="Signed  (2's comp)"  n_bits=64  bin_pt=0  preci_type=Single  exp_width=8  frac_width=24  assert_rate=off  rate_source=Explicitly  period=1  output_port=on  block_type=assert
  buscreate : Subsystem  AncestorBlock=casper_library_flow_control/bus_create  mask(bus_create){inputNum=2}
      mask prompts: inputNum "Number of inputs:"
      mask init:
      | bus_create_init(gcb,...
      |     'inputNum', inputNum);
  io_delay : Subsystem  AncestorBlock=casper_library_delays/pipeline  mask(pipeline){csp_latency=2}
      mask prompts: csp_latency "Latency"
      mask help:
      | An explicitly laid-out delay line to avoid mapping to SRL16s
      | for use in pipelining to help achieve timing closure.
      mask init:
      | pipeline_init(gcb,'latency',csp_latency);
      settings: AttributesFormatString=Latency = %<latency>
      mask Display:
      | port_label('input', 1, 'd');
      | port_label('output', 1, 'q');
      | disp(['Z^-', num2str(csp_latency)]);
  ss : Subsystem  Tag=casper:snapshot  AncestorBlock=casper_library_scopes/snapshot  mask(snapshot){storage=bram, dram_dimm=2, dram_clock=250, nsamples=14, data_width=128, offset=off, circap=off, value=off, ext_arm=off, ext_circ=off, provide_outputs=off, use_dsp48=on}
      mask prompts: storage "Storage medium"; dram_dimm "DRAM dimm"; dram_clock "DRAM clock rate"; nsamples "Number of Samples (2^?)"; data_width "Data width"; offset "Start delay support"; circap "Circular capture support"; value "Extra value capture support"; ext_arm "External arm support"; ext_circ "External circular capture support"; provide_outputs "Provide outputs"; use_dsp48 "Use DSP48s to implement counters"
      mask help:
      | Standard snap block, but with the following optional extras;
      |  1) Optionally delay the fabric trigger by a user-specified number of valids.
      |  2) Capture continuously after a trigger until a stop pulse is received. Data is captured into BRAM continuously, with old data being overwritten until a stop command is received. Then stop capturing when memory is filled. This enables you to get some data before and some data after the stop pulse. Use the 'tr_en_cnt' register to determine where you are in your vector. 'Addr' register's MSb now indicates 'busy capturing'.
      |  3) Optionally capture a value on an input port to a register at the same time as the first data sample.
      |  4) Implement counters using DSP48Es to save resources.
      mask init:
      | snapshot_init(gcb, ...
      |     'storage', storage, ...
      |     'dram_dimm', dram_dimm, ...
      |     'dram_clock', dram_clock, ...
      |     'nsamples', nsamples, ...
      |     'data_width', data_width, ...
      |     'offset', offset, ...
      |     'circap', circap, ...
      |     'value', value, ...
      |     'ext_arm', ext_arm, ...
      |     'ext_circ', ext_circ, ...
      |     'provide_outputs', 'off', ...
      |     'use_dsp48', use_dsp48);
      settings: AttributesFormatString=|
      | 128 wide, 16384 deep
      | debugID: 19954380
      mask TypeOptions storage: bram | dram
      mask Callback storage: snapshot_callback();
      mask TypeOptions dram_dimm: 1 | 2 | 3 | 4
      mask TypeOptions dram_clock: 200 | 250 | 266 | 300 | 333
      mask TypeOptions data_width: 8 | 16 | 32 | 64 | 128
  trig_delay : Subsystem  AncestorBlock=casper_library_delays/pipeline  mask(pipeline){csp_latency=2}
      mask prompts: csp_latency "Latency"
      mask help:
      | An explicitly laid-out delay line to avoid mapping to SRL16s
      | for use in pipelining to help achieve timing closure.
      mask init:
      | pipeline_init(gcb,'latency',csp_latency);
      settings: AttributesFormatString=Latency = %<latency>
      mask Display:
      | port_label('input', 1, 'd');
      | port_label('output', 1, 'q');
      | disp(['Z^-', num2str(csp_latency)]);
  we_delay : Subsystem  AncestorBlock=casper_library_delays/pipeline  mask(pipeline){csp_latency=2}
      mask prompts: csp_latency "Latency"
      mask help:
      | An explicitly laid-out delay line to avoid mapping to SRL16s
      | for use in pipelining to help achieve timing closure.
      mask init:
      | pipeline_init(gcb,'latency',csp_latency);
      settings: AttributesFormatString=Latency = %<latency>
      mask Display:
      | port_label('input', 1, 'd');
      | port_label('output', 1, 'q');
      | disp(['Z^-', num2str(csp_latency)]);
  arm_out : Outport
  wires:
  ss/1(arm_out) -> arm_out/1
  buscreate/1(bus_out) -> io_delay/1(d)
  io_delay/1(q) -> ss/1(din)
  in_m00/1 -> assert_m00/1
  assert_m00/1 -> buscreate/1(in1)
  in_m10/1 -> assert_m10/1
  assert_m10/1 -> buscreate/2(in2)
  we/1 -> we_delay/1(d)
  we_delay/1(q) -> ss/2(we)
  trig/1 -> trig_delay/1(d)
  trig_delay/1(q) -> ss/3(trig)

== system zcu216_tut_rfdc/counter_ctrl ==
  sim_1 : Inport
  convert1_1 : DataTypeConversion  OutDataTypeStr=fixdt('ufix32_En0')  LockScale=on
  convert2_1 : DataTypeConversion  OutDataTypeStr=fixdt('ufix32_En0')  ConvertRealWorld=Stored Integer (SI)  LockScale=on
  gain_1 : Gain
  io_delay : xbsIndex_r4/Delay  rst=off  infoeditControl=Selection of Reset will increase slice count due to use of real FFs and instead of SRLs  en=off  latency=0  reg_retiming=on  dbl_ovrd=off  block_type=delay
  reint1 : xbsIndex_r4/Reinterpret  force_arith_type=on  arith_type=Unsigned  force_bin_pt=on  bin_pt=0  block_type=reinterpret
  slice_reg : xbsIndex_r4/Slice  nbits=32  boolean_output=off  mode=Lower Bit Location + Width  bit1=0  base1=MSB of Input  bit0=0  base0=LSB of Input  dbl_ovrd=off  block_type=slice
  zcu216_tut_rfdc_counter_ctrl_user_data_out : xbsIndex_r4/Gateway In  gui_display_data_type=Fixed-point  arith_type=Unsigned  n_bits=32  bin_pt=0  preci_type=Single  exp_width=8  frac_width=24  rows=1  columns=1  quantization="Round  (unbiased: +/- Inf)"  overflow=Saturate  period=1  UseAsADC=off  ADCChannel='1'  interface=None  automatic_assignment=on  address_offset=hex2dec('00')  intf_name=''  intf_description=''  default_value=0  timing_constraint=None  locs_specified=off  LOCs={}  io_standard={}  inherit_from_input=off  hdl_port=on  dbl_ovrd=off  block_type=gatewayin
  in_reg : Outport  VectorParamsAs1DForOutWhenUnconnected=on
  wires:
  zcu216_tut_rfdc_counter_ctrl_user_data_out/1 -> io_delay/1
  sim_1/1 -> convert1_1/1
  convert1_1/1 -> convert2_1/1
  convert2_1/1 -> gain_1/1
  gain_1/1 -> zcu216_tut_rfdc_counter_ctrl_user_data_out/1
  io_delay/1 -> slice_reg/1
  slice_reg/1 -> reint1/1
  reint1/1 -> in_reg/1

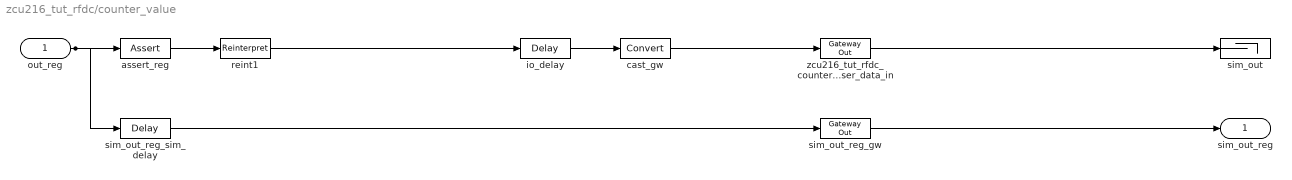
== system zcu216_tut_rfdc/counter_value ==
  out_reg : Inport
  assert_reg : xbsIndex_r4/Assert  assert_type=on  type_source=Explicitly  gui_display_data_type=Fixed-point  arith_type=Unsigned  n_bits=32  bin_pt=0  preci_type=Single  exp_width=8  frac_width=24  assert_rate=off  rate_source=Explicitly  period=1  output_port=on  block_type=assert
  cast_gw : xbsIndex_r4/Convert  gui_display_data_type=Fixed-point  arith_type=Unsigned  n_bits=32  bin_pt=0  float_type=Single  exp_bits=8  fraction_bits=24  quantization=Truncate  overflow=Wrap  en=off  latency=1  pipeline=off  dbl_ovrd=off  block_type=convert
  io_delay : xbsIndex_r4/Delay  rst=off  infoeditControl=Selection of Reset will increase slice count due to use of real FFs and instead of SRLs  en=off  latency=0  reg_retiming=on  dbl_ovrd=off  block_type=delay
  reint1 : xbsIndex_r4/Reinterpret  force_arith_type=on  arith_type=Unsigned  force_bin_pt=on  bin_pt=0  block_type=reinterpret
  sim_out : Terminator
  sim_out_reg_gw : xbsIndex_r4/Gateway Out  inherit_from_input=off  hdl_port=off  rows=1  columns=1  UseAsDAC=off  DACChannel='1'  interface=None  automatic_assignment=on  address_offset=hex2dec('00')  intf_name=''  intf_description=''  timing_constraint=None  locs_specified=off  LOCs={}  io_standard={}  block_type=gatewayout
  sim_out_reg_sim_delay : xbsIndex_r4/Delay  rst=off  infoeditControl=Selection of Reset will increase slice count due to use of real FFs and instead of SRLs  en=off  latency=1  reg_retiming=on  dbl_ovrd=off  block_type=delay
  zcu216_tut_rfdc_counter_value_user_data_in : xbsIndex_r4/Gateway Out  inherit_from_input=off  hdl_port=on  rows=1  columns=1  UseAsDAC=off  DACChannel='1'  interface=None  automatic_assignment=on  address_offset=hex2dec('00')  intf_name=''  intf_description=''  timing_constraint=None  locs_specified=off  LOCs={}  io_standard={}  block_type=gatewayout
  sim_out_reg : Outport  VectorParamsAs1DForOutWhenUnconnected=on
  wires:
  sim_out_reg_sim_delay/1 -> sim_out_reg_gw/1
  sim_out_reg_gw/1 -> sim_out_reg/1
  io_delay/1 -> cast_gw/1
  cast_gw/1 -> zcu216_tut_rfdc_counter_value_user_data_in/1
  zcu216_tut_rfdc_counter_value_user_data_in/1 -> sim_out/1
  out_reg/1 -> sim_out_reg_sim_delay/1, assert_reg/1
  assert_reg/1 -> reint1/1
  reint1/1 -> io_delay/1
